simulink subsystem "controlMapping"  (R2026a)
settings: Solver=VariableStepAuto
settings Model: Creator=maxhu  LastModifiedBy=maxhu

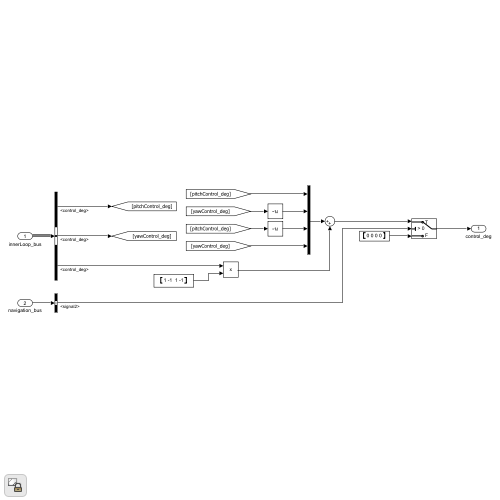
[thumbnail: Simulink's stored preview of the top-level diagram]
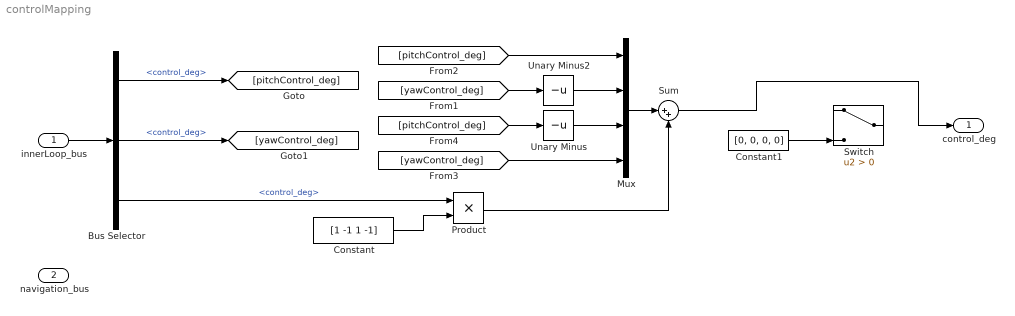
== system controlMapping ==
  innerLoop_bus : Inport
  navigation_bus : Inport  Port=2
  Bus Selector : BusSelector  OutputSignals=pitchInnerLoop_bus.control_deg,yawInnerLoop_bus.control_deg,rollInnerLoop_bus.control_deg
  Constant : Constant  Value=[1 -1 1 -1]
  Constant1 : Constant  Value=[0, 0, 0, 0]
  Mux : Mux
  Product : Product
  Sum : Sum  Inputs=|++
  Switch : Switch  Criteria=u2 > Threshold  SaturateOnIntegerOverflow=off  InputSameDT=off
  Unary Minus : UnaryMinus
  Unary Minus2 : UnaryMinus
  control_deg : Outport
  wires:
  [pitchControl_deg] -> Unary Minus/1
  Mux/1 -> Sum/1
  innerLoop_bus/1 -> Bus Selector/1
  [yawControl_deg] -> Unary Minus2/1
  Unary Minus2/1 -> Mux/2
  [yawControl_deg] -> Mux/4
  Bus Selector/1 -> [pitchControl_deg]  "<control_deg>"
  Bus Selector/2 -> [yawControl_deg]  "<control_deg>"
  Product/1 -> Sum/2
  Bus Selector/3 -> Product/1  "<control_deg>"
  Constant/1 -> Product/2
  [pitchControl_deg] -> Mux/1
  Unary Minus/1 -> Mux/3
  Constant1/1 -> Switch/3
  Sum/1 -> control_deg/1
